simulink model "casper_fft_xaui"  (Simulink 6.2)
settings: Solver=ode45  StartTime=0.0  StopTime=10.0  RelTol=1e-3
undefined symbols (not defined in the file): BEE2_usr
libraries: xbsIndex_r3 x68, xps_library x23, fft_library x3, adcscope_lib x3, delay_lib x2, correlator_library x1
settings Model: LastModifiedBy=lspitler
settings DebuggingCC: SolverPrmCheckMsg=warning

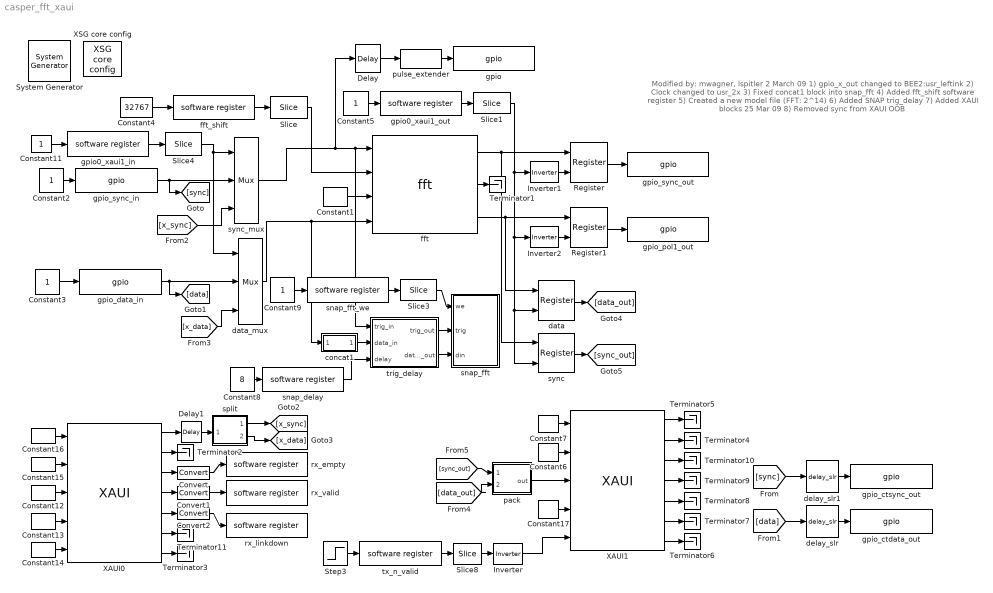
== system casper_fft_xaui ==
  note: Modified by: mwagner, lspitler
      | 2 March 09
      | 1) gpio_x_out changed to BEE2:usr_leftink
      | 2) Clock changed to usr_2x
      | 3) Fixed concat1 block into snap_fft
      | 4) Added fft_shift software register
      | 5) Created a new model file (FFT: 2^14)
      | 6) Added SNAP trig_delay
      | 7) Added XAUI blocks
      | 25 Mar 09
      | 8) Removed sync from XAUI OOB
  " System Generator" : xbsIndex_r3/ System Generator  Tag=genX  xilinxfamily=Virtex2P  part=xc2vp70  speed=-7  package=ff1704  synthesis_tool=XST  directory=./casper_fft_xaui/sysgen  testbench=off  simulink_period=1  sysclk_period=4.878  incr_netlist=off  trim_vbits=Everywhere in SubSystem  dbl_ovrd=According to Block Masks  core_generation=According to Block Masks  run_coregen=off  deprecated_control=off  eval_field=0
      settings: AttributesFormatString=System\nGenerator
  Constant1 : xbsIndex_r3/Constant  const=0  equ=P=C  arith_type=Unsigned  n_bits=30  bin_pt=0  opselect=C  inp2=PCIN>>17  opr=+  inp1=P  carry=CIN  iostate=0  explicit_period=on  period=1  dbl_ovrd=off
  Constant{2..3,5,9,11} (5 alike) : Constant
  Constant12 : xbsIndex_r3/Constant  const=0  equ=P=C  arith_type=Unsigned  n_bits=32  bin_pt=0  opselect=C  inp2=PCIN>>17  opr=+  inp1=P  carry=CIN  iostate=0  explicit_period=on  period=1  dbl_ovrd=off
  Constant13 : xbsIndex_r3/Constant  const=0  equ=P=C  arith_type=Unsigned  n_bits=4  bin_pt=0  opselect=C  inp2=PCIN>>17  opr=+  inp1=P  carry=CIN  iostate=0  explicit_period=on  period=1  dbl_ovrd=off
  Constant14 : xbsIndex_r3/Constant  const=0  equ=P=C  arith_type=Boolean  n_bits=1  bin_pt=0  opselect=C  inp2=PCIN>>17  opr=+  inp1=P  carry=CIN  iostate=0  explicit_period=on  period=1  dbl_ovrd=off
  Constant15 : xbsIndex_r3/Constant  const=0  equ=P=C  arith_type=Boolean  n_bits=32  bin_pt=0  opselect=C  inp2=PCIN>>17  opr=+  inp1=P  carry=CIN  iostate=0  explicit_period=on  period=1  dbl_ovrd=off
  Constant16 : xbsIndex_r3/Constant  const=1  equ=P=C  arith_type=Boolean  n_bits=32  bin_pt=0  opselect=C  inp2=PCIN>>17  opr=+  inp1=P  carry=CIN  iostate=0  explicit_period=on  period=1  dbl_ovrd=off
  Constant17 : xbsIndex_r3/Constant  const=0  equ=P=C  arith_type=Unsigned  n_bits=4  bin_pt=0  opselect=C  inp2=PCIN>>17  opr=+  inp1=P  carry=CIN  iostate=0  explicit_period=on  period=1  dbl_ovrd=off
  Constant4 : Constant  Value=32767
  Constant6 : xbsIndex_r3/Constant  const=0  equ=P=C  arith_type=Boolean  n_bits=36  bin_pt=0  opselect=C  inp2=PCIN>>17  opr=+  inp1=P  carry=CIN  iostate=0  explicit_period=on  period=1  dbl_ovrd=off
  Constant7 : xbsIndex_r3/Constant  const=1  equ=P=C  arith_type=Boolean  n_bits=36  bin_pt=0  opselect=C  inp2=PCIN>>17  opr=+  inp1=P  carry=CIN  iostate=0  explicit_period=on  period=1  dbl_ovrd=off
  Constant8 : Constant  Value=8
  Convert : xbsIndex_r3/Convert  arith_type=Unsigned  n_bits=32  bin_pt=0  quantization=Truncate  overflow=Wrap  latency=0  explicit_period=on  period=1  dbl_ovrd=off  show_param=off  inserted_by_tool=off  pipeline=off
      settings: xl_area=[0, 0, 0, 0, 0, 0, 0]
  Convert1 : xbsIndex_r3/Convert  arith_type=Unsigned  n_bits=32  bin_pt=0  quantization=Truncate  overflow=Wrap  latency=0  explicit_period=on  period=1  dbl_ovrd=off  show_param=off  inserted_by_tool=off  pipeline=off
      settings: xl_area=[0, 0, 0, 0, 0, 0, 0]
  Convert2 : xbsIndex_r3/Convert  arith_type=Unsigned  n_bits=32  bin_pt=0  quantization=Truncate  overflow=Wrap  latency=0  explicit_period=on  period=1  dbl_ovrd=off  show_param=off  inserted_by_tool=off  pipeline=off
      settings: xl_area=[0, 0, 0, 0, 0, 0, 0]
  Delay : xbsIndex_r3/Delay  latency=1  reg_retiming=off  explicit_period=off  period=1  en=off  accept_only_valid=off  init_zero=on  dbl_ovrd=off  show_param=off
      settings: xl_area=[0, 0, 0, 0, 0, 0, 0]
  Delay1 : xbsIndex_r3/Delay  latency=1  reg_retiming=off  explicit_period=on  period=1  en=off  accept_only_valid=off  init_zero=on  dbl_ovrd=off  show_param=off
      settings: xl_area=[0, 0, 0, 0, 0, 0, 0]
  Inverter : xbsIndex_r3/Inverter  latency=0  explicit_period=off  period=1  en=off  dbl_ovrd=off  show_param=off
      settings: xl_area=[0, 0, 0, 0, 0, 0, 0]
  Inverter1 : xbsIndex_r3/Inverter  latency=0  explicit_period=off  period=1  en=off  dbl_ovrd=off  show_param=off
      settings: xl_area=[0, 0, 0, 0, 0, 0, 0]
  Inverter2 : xbsIndex_r3/Inverter  latency=0  explicit_period=off  period=1  en=off  dbl_ovrd=off  show_param=off
      settings: xl_area=[0, 0, 0, 0, 0, 0, 0]
  Register : xbsIndex_r3/Register  init=0  reg_only_valid=off  explicit_period=off  period=1  rst=off  en=on  out_en=off  dbl_ovrd=off  show_param=off
      settings: xl_area=[0, 0, 0, 0, 0, 0, 0]
  Register1 : xbsIndex_r3/Register  init=0  reg_only_valid=off  explicit_period=off  period=1  rst=off  en=on  out_en=off  dbl_ovrd=off  show_param=off
      settings: xl_area=[0, 0, 0, 0, 0, 0, 0]
  Slice : xbsIndex_r3/Slice  mode=Lower Bit Location + Width  nbits=15  bit1=0  base1=MSB of Input  bit0=0  base0=LSB of Input  boolean_output=off  explicit_period=off  period=1  dbl_ovrd=off
  Slice1 : xbsIndex_r3/Slice  mode=Lower Bit Location + Width  nbits=1  bit1=0  base1=MSB of Input  bit0=0  base0=LSB of Input  boolean_output=on  explicit_period=on  period=1  dbl_ovrd=off
  Slice3 : xbsIndex_r3/Slice  mode=Lower Bit Location + Width  nbits=1  bit1=0  base1=MSB of Input  bit0=0  base0=LSB of Input  boolean_output=on  explicit_period=on  period=1  dbl_ovrd=off
  Slice4 : xbsIndex_r3/Slice  mode=Lower Bit Location + Width  nbits=1  bit1=0  base1=MSB of Input  bit0=0  base0=LSB of Input  boolean_output=off  explicit_period=off  period=1  dbl_ovrd=off
  Slice8 : xbsIndex_r3/Slice  mode=Lower Bit Location + Width  nbits=1  bit1=0  base1=MSB of Input  bit0=0  base0=LSB of Input  boolean_output=on  explicit_period=on  period=1  dbl_ovrd=off
  Step3 : Step  SampleTime=0
  Terminator{1..11} (11 alike) : Terminator
  XAUI0 : xps_library/XAUI  Tag=xps:xaui  demux=2  port=BEE2_usr:0  show_param=off  pre_emph=3  swing=800
  XAUI1 : xps_library/XAUI  Tag=xps:xaui  demux=2  port=BEE2_usr:1  show_param=off  pre_emph=3  swing=800
  XSG core config : xps_library/XSG core config  Tag=xps:xsg  hw_sys=BEE2_usr  ibob_linux=off  clk_src=usr_clk2x  gpio_clk_io_group=iBOB:sma  gpio_clk_bit_index=0  clk_rate=205  sample_period=1  synthesis_tool=XST  mpc_type=powerpc405
  concat1 : Subsystem
  data : xbsIndex_r3/Register  init=0  reg_only_valid=off  explicit_period=off  period=1  rst=off  en=on  out_en=off  dbl_ovrd=off  show_param=off
      settings: xl_area=[0, 0, 0, 0, 0, 0, 0]
  data_mux : xbsIndex_r3/Mux  inputs=2  precision=Full  arith_type="Signed  (2's comp)"  n_bits=8  bin_pt=2  quantization=Truncate  overflow=Wrap  latency=2  explicit_period=on  period=1  en=off  dbl_ovrd=off  show_param=off  mux_type=off  use_rpm=off  gen_core=off
      settings: xl_area=[0, 0, 0, 0, 0, 0, 0]
  delay_slr : delay_lib/delay_slr  DelayLen=2048
  delay_slr1 : delay_lib/delay_slr  DelayLen=2048
  fft : fft_library/fft  FFTSize=15  BitWidth=18  n_inputs=0  quantization=Truncate  overflow=Wrap  add_latency=1  mult_latency=3  bram_latency=2
  fft_shift : xps_library/software register  Tag=xps:sw_reg  io_dir=From Processor  arith_type=Unsigned  bitwidth=32  bin_pt=0  sample_period=1  gw_name=casper_fft_xaui_fft_shift_user_data_out
  gpio : xps_library/gpio  Tag=xps:gpio  io_group=BEE2_usr:led  io_dir=out  arith_type=Boolean  bitwidth=1  bin_pt=0  bit_index=0  sample_period=1  use_single_ended=off  use_ddr=off  reg_iob=on  reg_clk_phase=0  termination=None
  gpio0_xaui1_in : xps_library/software register  Tag=xps:sw_reg  io_dir=From Processor  arith_type=Unsigned  bitwidth=32  bin_pt=0  sample_period=1  gw_name=casper_fft_xaui_gpio0_xaui1_in_user_data_out
  gpio0_xaui1_out : xps_library/software register  Tag=xps:sw_reg  io_dir=From Processor  arith_type=Unsigned  bitwidth=32  bin_pt=0  sample_period=1  gw_name=casper_fft_xaui_gpio0_xaui1_out_user_data_out
  gpio_ctdata_out : xps_library/gpio  Tag=xps:gpio  io_group=BEE2_usr:leftlink  io_dir=out  arith_type=Unsigned  bitwidth=36  bin_pt=0  bit_index=[0:35]  sample_period=1  use_single_ended=off  use_ddr=off  reg_iob=on  reg_clk_phase=0  termination=None
  gpio_ctsync_out : xps_library/gpio  Tag=xps:gpio  io_group=BEE2_usr:leftlink  io_dir=out  arith_type=Boolean  bitwidth=1  bin_pt=0  bit_index=36  sample_period=1  use_single_ended=off  use_ddr=off  reg_iob=on  reg_clk_phase=0  termination=None
  gpio_data_in : xps_library/gpio  Tag=xps:gpio  io_group=BEE2_usr:rightlink  io_dir=in  arith_type=Unsigned  bitwidth=36  bin_pt=0  bit_index=[37:72]  sample_period=1  use_single_ended=off  use_ddr=off  reg_iob=on  reg_clk_phase=0  termination=None
  gpio_pol1_out : xps_library/gpio  Tag=xps:gpio  io_group=BEE2_usr:leftlink  io_dir=out  arith_type=Unsigned  bitwidth=36  bin_pt=0  bit_index=[37:72]  sample_period=1  use_single_ended=off  use_ddr=off  reg_iob=on  reg_clk_phase=0  termination=None
  gpio_sync_in : xps_library/gpio  Tag=xps:gpio  io_group=BEE2_usr:rightlink  io_dir=in  arith_type=Boolean  bitwidth=1  bin_pt=0  bit_index=73  sample_period=1  use_single_ended=off  use_ddr=off  reg_iob=on  reg_clk_phase=0  termination=None
  gpio_sync_out : xps_library/gpio  Tag=xps:gpio  io_group=BEE2_usr:leftlink  io_dir=out  arith_type=Boolean  bitwidth=1  bin_pt=0  bit_index=73  sample_period=1  use_single_ended=off  use_ddr=off  reg_iob=on  reg_clk_phase=0  termination=None
  pack : Subsystem
  pulse_extender : adcscope_lib/pulse_extender  pulse_len=2^25
  rx_empty : xps_library/software register  Tag=xps:sw_reg  io_dir=To Processor  arith_type=Unsigned  bitwidth=32  bin_pt=0  sample_period=1  gw_name=casper_fft_xaui_rx_empty_user_data_in
  rx_linkdown : xps_library/software register  Tag=xps:sw_reg  io_dir=To Processor  arith_type=Unsigned  bitwidth=32  bin_pt=0  sample_period=1  gw_name=casper_fft_xaui_rx_linkdown_user_data_in
  rx_valid : xps_library/software register  Tag=xps:sw_reg  io_dir=To Processor  arith_type=Unsigned  bitwidth=32  bin_pt=0  sample_period=1  gw_name=casper_fft_xaui_rx_valid_user_data_in
  snap_delay : xps_library/software register  Tag=xps:sw_reg  io_dir=From Processor  arith_type=Unsigned  bitwidth=32  bin_pt=0  sample_period=1  gw_name=casper_fft_xaui_snap_delay_user_data_out
  snap_fft : Subsystem  mask{nsamples=12}
      mask prompts: nsamples "number of samples (2^?)"
  snap_fft_we : xps_library/software register  Tag=xps:sw_reg  io_dir=From Processor  arith_type=Unsigned  bitwidth=32  bin_pt=0  sample_period=1  gw_name=casper_fft_xaui_snap_fft_we_user_data_out
  split : Subsystem
  sync : xbsIndex_r3/Register  init=0  reg_only_valid=off  explicit_period=off  period=1  rst=off  en=on  out_en=off  dbl_ovrd=off  show_param=off
      settings: xl_area=[0, 0, 0, 0, 0, 0, 0]
  sync_mux : xbsIndex_r3/Mux  inputs=2  precision=Full  arith_type="Signed  (2's comp)"  n_bits=8  bin_pt=2  quantization=Truncate  overflow=Wrap  latency=2  explicit_period=on  period=1  en=off  dbl_ovrd=off  show_param=off  mux_type=off  use_rpm=off  gen_core=off
      settings: xl_area=[0, 0, 0, 0, 0, 0, 0]
  trig_delay : Subsystem
  tx_n_valid : xps_library/software register  Tag=xps:sw_reg  io_dir=From Processor  arith_type=Unsigned  bitwidth=32  bin_pt=0  sample_period=1  gw_name=casper_fft_xaui_tx_n_valid_user_data_out
  wires:
  fft_shift/1 -> Slice/1
  Constant1/1 -> fft/3
  Constant2/1 -> gpio_sync_in/1
  Constant3/1 -> gpio_data_in/1
  snap_fft_we/1 -> Slice3/1
  Slice3/1 -> snap_fft/1(we)
  Constant9/1 -> snap_fft_we/1
  pulse_extender/1 -> gpio/1
  Constant4/1 -> fft_shift/1
  Slice/1 -> fft/2
  trig_delay/1(trig_out) -> snap_fft/2(trig)
  trig_delay/2(data_out) -> snap_fft/3(din)
  concat1/1(Out1) -> trig_delay/2(data_in)
  fft/1 -> Register/1, sync/1
  fft/3 -> Register1/1, data/1
  Inverter1/1 -> Register/2
  Inverter2/1 -> Register1/2
  Register/1 -> gpio_sync_out/1
  Register1/1 -> gpio_pol1_out/1
  Constant5/1 -> gpio0_xaui1_out/1
  gpio0_xaui1_out/1 -> Slice1/1
  Slice1/1 -> Inverter1/1, Inverter2/1, data/2, sync/2
  Constant6/1 -> XAUI1/2
  Constant7/1 -> XAUI1/1
  XAUI1/2 -> Terminator4/1
  XAUI1/6 -> Terminator7/1
  XAUI1/7 -> Terminator6/1
  XAUI1/3 -> Terminator10/1
  XAUI1/4 -> Terminator9/1
  XAUI1/5 -> Terminator8/1
  tx_n_valid/1 -> Slice8/1
  Step3/1 -> tx_n_valid/1
  Slice8/1 -> Inverter/1
  XAUI1/1 -> Terminator5/1
  delay_slr1/1 -> gpio_ctsync_out/1
  delay_slr/1 -> gpio_ctdata_out/1
  gpio_sync_in/1 -> sync_mux/2, [sync]
  sync_mux/1 -> fft/1, trig_delay/1(trig_in), Delay/1
  gpio_data_in/1 -> data_mux/2, [data]
  XAUI0/2 -> Terminator2/1
  data_mux/1 -> fft/4, concat1/1(In1)
  XAUI0/1 -> Delay1/1
  gpio0_xaui1_in/1 -> Slice4/1
  Constant11/1 -> gpio0_xaui1_in/1
  Convert/1 -> rx_empty/1
  Convert1/1 -> rx_valid/1
  Convert2/1 -> rx_linkdown/1
  XAUI0/3 -> Convert/1
  XAUI0/4 -> Convert1/1
  XAUI0/5 -> Convert2/1
  Constant12/1 -> XAUI0/3
  Constant13/1 -> XAUI0/4
  Constant14/1 -> XAUI0/5
  Constant15/1 -> XAUI0/2
  Constant16/1 -> XAUI0/1
  Slice4/1 -> sync_mux/1, data_mux/1
  [sync] -> delay_slr1/1
  [data] -> delay_slr/1
  Constant8/1 -> snap_delay/1
  snap_delay/1 -> trig_delay/3(delay)
  Delay/1 -> pulse_extender/1
  fft/2 -> Terminator1/1
  Delay1/1 -> split/1(In1)
  split/1(sync) -> [x_sync]
  split/2(data) -> [x_data]
  [x_sync] -> sync_mux/3
  [x_data] -> data_mux/3
  Constant17/1 -> XAUI1/4
  XAUI0/6 -> Terminator11/1
  XAUI0/7 -> Terminator3/1
  data/1 -> [data_out]
  pack/1(out) -> XAUI1/3
  sync/1 -> [sync_out]
  Inverter/1 -> XAUI1/5
  [sync_out] -> pack/1(sync)
  [data_out] -> pack/2(data)

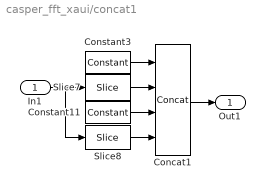
== system casper_fft_xaui/concat1 ==
  In1 : Inport  Port=1  LatchInput=off
  Concat1 : xbsIndex_r3/Concat  num_inputs=4  explicit_period=on  period=1  dbl_ovrd=off
  Constant11 : xbsIndex_r3/Constant  const=0  equ=P=C  arith_type=Unsigned  n_bits=14  bin_pt=0  opselect=C  inp2=PCIN>>17  opr=+  inp1=P  carry=CIN  iostate=0  explicit_period=on  period=1  dbl_ovrd=off
  Constant3 : xbsIndex_r3/Constant  const=0  equ=P=C  arith_type=Unsigned  n_bits=14  bin_pt=0  opselect=C  inp2=PCIN>>17  opr=+  inp1=P  carry=CIN  iostate=0  explicit_period=on  period=1  dbl_ovrd=off
  Slice7 : xbsIndex_r3/Slice  mode=Upper Bit Location + Width  nbits=18  bit1=0  base1=MSB of Input  bit0=0  base0=LSB of Input  boolean_output=off  explicit_period=on  period=1  dbl_ovrd=off
  Slice8 : xbsIndex_r3/Slice  mode=Lower Bit Location + Width  nbits=18  bit1=0  base1=MSB of Input  bit0=0  base0=LSB of Input  boolean_output=off  explicit_period=on  period=1  dbl_ovrd=off
  Out1 : Outport
  wires:
  Slice7/1 -> Concat1/2
  Slice8/1 -> Concat1/4
  Constant3/1 -> Concat1/1
  Constant11/1 -> Concat1/3
  In1/1 -> Slice7/1, Slice8/1
  Concat1/1 -> Out1/1

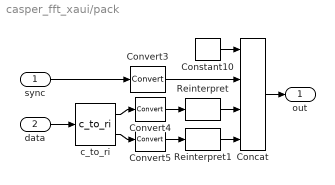
== system casper_fft_xaui/pack ==
  sync : Inport  Port=1  LatchInput=off
  data : Inport  Port=2  LatchInput=off
  Concat : xbsIndex_r3/Concat  num_inputs=4  explicit_period=on  period=1  dbl_ovrd=off
  Constant10 : xbsIndex_r3/Constant  const=0  equ=P=C  arith_type=Unsigned  n_bits=1  bin_pt=0  opselect=C  inp2=PCIN>>17  opr=+  inp1=P  carry=CIN  iostate=0  explicit_period=on  period=1  dbl_ovrd=off
  Convert3 : xbsIndex_r3/Convert  arith_type=Unsigned  n_bits=1  bin_pt=0  quantization=Truncate  overflow=Wrap  latency=1  explicit_period=on  period=1  dbl_ovrd=off  show_param=off  inserted_by_tool=off  pipeline=off
      settings: xl_area=[0, 0, 0, 0, 0, 0, 0]
  Convert4 : xbsIndex_r3/Convert  arith_type="Signed  (2's comp)"  n_bits=15  bin_pt=14  quantization=Truncate  overflow=Wrap  latency=1  explicit_period=on  period=1  dbl_ovrd=off  show_param=off  inserted_by_tool=off  pipeline=off
      settings: xl_area=[0, 0, 0, 0, 0, 0, 0]
  Convert5 : xbsIndex_r3/Convert  arith_type="Signed  (2's comp)"  n_bits=15  bin_pt=14  quantization=Truncate  overflow=Wrap  latency=1  explicit_period=on  period=1  dbl_ovrd=off  show_param=off  inserted_by_tool=off  pipeline=off
      settings: xl_area=[0, 0, 0, 0, 0, 0, 0]
  Reinterpret : xbsIndex_r3/Reinterpret  force_arith_type=on  arith_type=Unsigned  force_bin_pt=on  bin_pt=0  force_valid=on
  Reinterpret1 : xbsIndex_r3/Reinterpret  force_arith_type=on  arith_type=Unsigned  force_bin_pt=on  bin_pt=0  force_valid=on
  c_to_ri : fft_library/c_to_ri  BitWidth=18
  out : Outport
  wires:
  Reinterpret1/1 -> Concat/4
  Convert5/1 -> Reinterpret1/1
  data/1 -> c_to_ri/1
  Concat/1 -> out/1
  sync/1 -> Convert3/1
  Reinterpret/1 -> Concat/3
  Convert4/1 -> Reinterpret/1
  Convert3/1 -> Concat/2
  c_to_ri/2 -> Convert5/1
  c_to_ri/1 -> Convert4/1
  Constant10/1 -> Concat/1

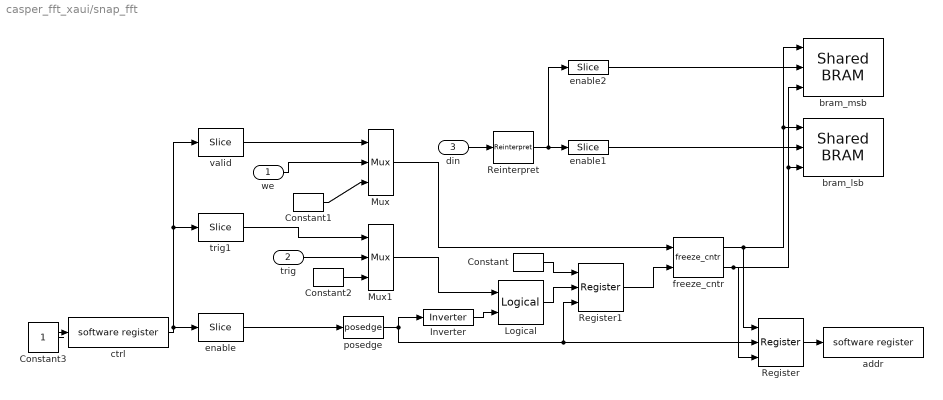
== system casper_fft_xaui/snap_fft ==
  we : Inport  Port=1  LatchInput=off
  trig : Inport  Port=2  LatchInput=off
  din : Inport  Port=3  LatchInput=off
  Constant : xbsIndex_r3/Constant  const=1  equ=P=C  arith_type=Boolean  n_bits=1  bin_pt=0  opselect=C  inp2=PCIN>>17  opr=+  inp1=P  carry=CIN  iostate=0  explicit_period=on  period=1  dbl_ovrd=off
  Constant1 : xbsIndex_r3/Constant  const=1  equ=P=C  arith_type=Boolean  n_bits=1  bin_pt=0  opselect=C  inp2=PCIN>>17  opr=+  inp1=P  carry=CIN  iostate=0  explicit_period=on  period=1  dbl_ovrd=off
  Constant2 : xbsIndex_r3/Constant  const=1  equ=P=C  arith_type=Boolean  n_bits=1  bin_pt=0  opselect=C  inp2=PCIN>>17  opr=+  inp1=P  carry=CIN  iostate=0  explicit_period=on  period=1  dbl_ovrd=off
  Constant3 : Constant
  Inverter : xbsIndex_r3/Inverter  latency=0  explicit_period=on  period=1  en=off  dbl_ovrd=off  show_param=off
      settings: xl_area=[0, 0, 0, 0, 0, 0, 0]
  Logical : xbsIndex_r3/Logical  logical_function=AND  inputs=2  precision=Full  arith_type=Unsigned  n_bits=8  bin_pt=2  align_bp=on  latency=0  explicit_period=off  period=1  en=off  dbl_ovrd=off  show_param=off
      settings: xl_area=[0, 0, 0, 0, 0, 0, 0]
  Mux : xbsIndex_r3/Mux  inputs=2  precision=Full  arith_type="Signed  (2's comp)"  n_bits=8  bin_pt=2  quantization=Truncate  overflow=Wrap  latency=0  explicit_period=on  period=1  en=off  dbl_ovrd=off  show_param=off  mux_type=off  use_rpm=off  gen_core=off
      settings: xl_area=[0, 0, 0, 0, 0, 0, 0]
  Mux1 : xbsIndex_r3/Mux  inputs=2  precision=Full  arith_type="Signed  (2's comp)"  n_bits=8  bin_pt=2  quantization=Truncate  overflow=Wrap  latency=0  explicit_period=on  period=1  en=off  dbl_ovrd=off  show_param=off  mux_type=off  use_rpm=off  gen_core=off
      settings: xl_area=[0, 0, 0, 0, 0, 0, 0]
  Register : xbsIndex_r3/Register  init=0  reg_only_valid=off  explicit_period=on  period=1  rst=on  en=on  out_en=off  dbl_ovrd=off  show_param=off
      settings: xl_area=[0, 0, 0, 0, 0, 0, 0]
  Register1 : xbsIndex_r3/Register  init=0  reg_only_valid=off  explicit_period=on  period=1  rst=on  en=on  out_en=off  dbl_ovrd=off  show_param=off
      settings: xl_area=[0, 0, 0, 0, 0, 0, 0]
  Reinterpret : xbsIndex_r3/Reinterpret  force_arith_type=on  arith_type=Unsigned  force_bin_pt=on  bin_pt=0  force_valid=on
  addr : xps_library/software register  Tag=xps:sw_reg  io_dir=To Processor  arith_type=Unsigned  bitwidth=32  bin_pt=0  sample_period=1  gw_name=casper_fft_xaui_snap_fft_addr_user_data_in
  bram_lsb : xps_library/Shared BRAM  Tag=xps:bram  arith_type=Unsigned  addr_width=nsamples  data_width=32  data_bin_pt=0  init_vals=0  sample_rate=1
  bram_msb : xps_library/Shared BRAM  Tag=xps:bram  arith_type=Unsigned  addr_width=nsamples  data_width=32  data_bin_pt=0  init_vals=0  sample_rate=1
  ctrl : xps_library/software register  Tag=xps:sw_reg  io_dir=From Processor  arith_type=Unsigned  bitwidth=32  bin_pt=0  sample_period=1  gw_name=casper_fft_xaui_snap_fft_ctrl_user_data_out
  enable : xbsIndex_r3/Slice  mode=Lower Bit Location + Width  nbits=1  bit1=0  base1=MSB of Input  bit0=0  base0=LSB of Input  boolean_output=on  explicit_period=on  period=1  dbl_ovrd=off
  enable1 : xbsIndex_r3/Slice  mode=Lower Bit Location + Width  nbits=32  bit1=0  base1=MSB of Input  bit0=0  base0=LSB of Input  boolean_output=off  explicit_period=on  period=1  dbl_ovrd=off
  enable2 : xbsIndex_r3/Slice  mode=Lower Bit Location + Width  nbits=32  bit1=0  base1=MSB of Input  bit0=32  base0=LSB of Input  boolean_output=off  explicit_period=on  period=1  dbl_ovrd=off
  freeze_cntr : correlator_library/freeze_cntr  CounterBits=nsamples
  posedge : adcscope_lib/posedge  Tag=Rising Edge Detector  yummy=on
  trig1 : xbsIndex_r3/Slice  mode=Lower Bit Location + Width  nbits=1  bit1=1  base1=MSB of Input  bit0=1  base0=LSB of Input  boolean_output=on  explicit_period=on  period=1  dbl_ovrd=off
  valid : xbsIndex_r3/Slice  mode=Lower Bit Location + Width  nbits=1  bit1=0  base1=MSB of Input  bit0=2  base0=LSB of Input  boolean_output=on  explicit_period=on  period=1  dbl_ovrd=off
  wires:
  Constant3/1 -> ctrl/1
  ctrl/1 -> valid/1, trig1/1, enable/1
  valid/1 -> Mux/1
  trig1/1 -> Mux1/1
  freeze_cntr/2 -> bram_msb/3, bram_lsb/3, Register/3
  freeze_cntr/1 -> Register/1, bram_msb/1, bram_lsb/1
  Mux/1 -> freeze_cntr/1
  Mux1/1 -> Logical/1
  Constant/1 -> Register1/1
  Logical/1 -> Register1/2
  Register1/1 -> freeze_cntr/2
  Inverter/1 -> Logical/2
  din/1 -> Reinterpret/1
  Constant2/1 -> Mux1/3
  Constant1/1 -> Mux/3
  trig/1 -> Mux1/2
  we/1 -> Mux/2
  Reinterpret/1 -> enable2/1, enable1/1
  enable1/1 -> bram_lsb/2
  enable2/1 -> bram_msb/2
  Register/1 -> addr/1
  posedge/1 -> Register1/3, Register/2, Inverter/1
  enable/1 -> posedge/1

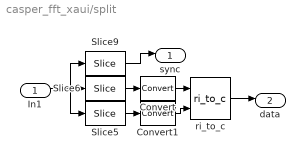
== system casper_fft_xaui/split ==
  In1 : Inport  Port=1  LatchInput=off
  Convert : xbsIndex_r3/Convert  arith_type="Signed  (2's comp)"  n_bits=18  bin_pt=17  quantization=Truncate  overflow=Wrap  latency=0  explicit_period=on  period=1  dbl_ovrd=off  show_param=off  inserted_by_tool=off  pipeline=off
      settings: xl_area=[0, 0, 0, 0, 0, 0, 0]
  Convert1 : xbsIndex_r3/Convert  arith_type="Signed  (2's comp)"  n_bits=18  bin_pt=17  quantization=Truncate  overflow=Wrap  latency=0  explicit_period=on  period=1  dbl_ovrd=off  show_param=off  inserted_by_tool=off  pipeline=off
      settings: xl_area=[0, 0, 0, 0, 0, 0, 0]
  Slice5 : xbsIndex_r3/Slice  mode=Lower Bit Location + Width  nbits=15  bit1=0  base1=MSB of Input  bit0=0  base0=LSB of Input  boolean_output=off  explicit_period=on  period=1  dbl_ovrd=off
  Slice6 : xbsIndex_r3/Slice  mode=Lower Bit Location + Width  nbits=15  bit1=0  base1=MSB of Input  bit0=15  base0=LSB of Input  boolean_output=off  explicit_period=on  period=1  dbl_ovrd=off
  Slice9 : xbsIndex_r3/Slice  mode=Lower Bit Location + Width  nbits=1  bit1=0  base1=MSB of Input  bit0=30  base0=LSB of Input  boolean_output=on  explicit_period=on  period=1  dbl_ovrd=off
  ri_to_c : fft_library/ri_to_c  likes_cookies=off
  sync : Outport
  data : Outport  Port=2
  wires:
  In1/1 -> Slice5/1, Slice6/1, Slice9/1
  Slice6/1 -> Convert/1
  Slice5/1 -> Convert1/1
  Convert/1 -> ri_to_c/1
  Convert1/1 -> ri_to_c/2
  Slice9/1 -> sync/1
  ri_to_c/1 -> data/1

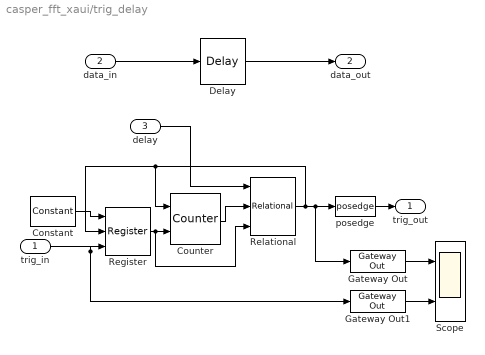
== system casper_fft_xaui/trig_delay ==
  trig_in : Inport  Port=1  LatchInput=off
  data_in : Inport  Port=2  LatchInput=off
  delay : Inport  Port=3  LatchInput=off
  Constant : xbsIndex_r3/Constant  const=1  equ=P=C  arith_type=Boolean  n_bits=32  bin_pt=0  opselect=C  inp2=PCIN>>17  opr=+  inp1=P  carry=CIN  iostate=0  explicit_period=on  period=1  dbl_ovrd=off
  Counter : xbsIndex_r3/Counter  cnt_type=Free Running  n_bits=32  bin_pt=0  arith_type=Unsigned  start_count=0  cnt_to=Inf  cnt_by_val=1  operation=Up  explicit_period=on  period=1  load_pin=off  rst=on  en=on  dbl_ovrd=off  show_param=off  use_rpm=on  gen_core=off
      settings: xl_area=[0, 0, 0, 0, 0, 0, 0]
  Delay : xbsIndex_r3/Delay  latency=2  reg_retiming=off  explicit_period=on  period=1  en=off  accept_only_valid=off  init_zero=on  dbl_ovrd=off  show_param=off
      settings: xl_area=[0, 0, 0, 0, 0, 0, 0]
  Gateway Out : xbsIndex_r3/Gateway Out  output_type=Double  nbits=8  bin_pt=6  arith_type=Boolean  quantization=Truncate  overflow=Wrap  hdl_port=on  timing_constraint=None  locs_specified=off  LOCs={}  needs_fixed_name=off  show_param=off
      settings: xl_area=[0, 0, 0, 0, 0, 0, 0]
  Gateway Out1 : xbsIndex_r3/Gateway Out  output_type=Double  nbits=8  bin_pt=6  arith_type=Boolean  quantization=Truncate  overflow=Wrap  hdl_port=on  timing_constraint=None  locs_specified=off  LOCs={}  needs_fixed_name=off  show_param=off
      settings: xl_area=[0, 0, 0, 0, 0, 0, 0]
  Register : xbsIndex_r3/Register  init=0  reg_only_valid=off  explicit_period=on  period=1  rst=on  en=on  out_en=off  dbl_ovrd=off  show_param=off
      settings: xl_area=[0, 0, 0, 0, 0, 0, 0]
  Relational : xbsIndex_r3/Relational  mode=a=b  latency=1  explicit_period=on  period=1  en=on  dbl_ovrd=off  show_param=off
      settings: xl_area=[0, 0, 0, 0, 0, 0, 0]
  Scope : Scope  NumInputPorts=2
      settings: YMin=-5~-5  YMax=5~5
  posedge : adcscope_lib/posedge  Tag=Rising Edge Detector  yummy=on
  trig_out : Outport
  data_out : Outport  Port=2
  wires:
  delay/1 -> Relational/1
  trig_in/1 -> Register/3, Gateway Out1/1
  Constant/1 -> Register/1
  Relational/1 -> Register/2, Counter/1, Gateway Out/1, posedge/1
  Register/1 -> Counter/2, Relational/3
  Counter/1 -> Relational/2
  Gateway Out/1 -> Scope/1
  Gateway Out1/1 -> Scope/2
  data_in/1 -> Delay/1
  Delay/1 -> data_out/1
  posedge/1 -> trig_out/1
